simulink subsystem "acq_block"  (R2019b)
settings: Solver=VariableStepAuto  StartTime=0.0  StopTime=10.0  RelTol=1e-3
undefined symbols (not defined in the file): fs, Len, Radix
libraries: commseqgen3 x2, dspstat3 x2, dspsigops x2, dspxfrm3 x1
settings Model: Creator=nishantmittal  LastModifiedBy=nishantmittal

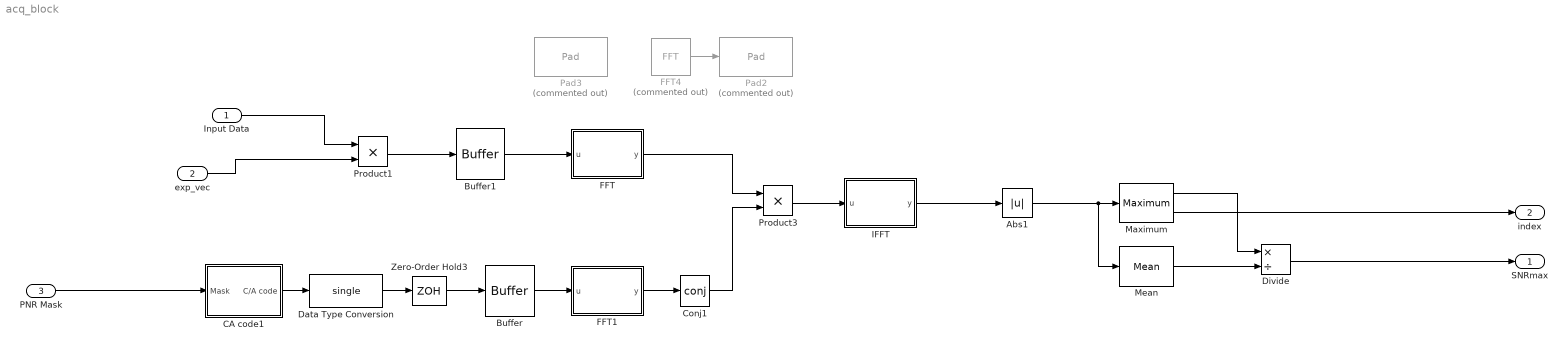
== system acq_block ==
  "Input Data " : Inport
  exp_vec : Inport  Port=2
  PNR Mask : Inport  Port=3
  Abs1 : Abs
  Buffer : Buffer  N=Len  ic=1  OutputFrames=off
  Buffer1 : Buffer  N=Len  ic=1  OutputFrames=off
  CA code1 : Subsystem
  Conj1 : Math  Operator=conj  SignedPower=off  SaturateOnIntegerOverflow=on
  Data Type Conversion : DataTypeConversion  OutDataTypeStr=single
  Divide : Product  Inputs=*/
  FFT : MATLAB Function  TreatAsAtomicUnit=on
  FFT1 : MATLAB Function  TreatAsAtomicUnit=on
  FFT4 : dspxfrm3/FFT  Commented=on  FFTImplementation=Radix-2  CompMethod=Table lookup  TableOpt=NEW  TableOptActive=Speed  BitRevOrder=off  Normalize=off  InheritFFTLength=off  FFTLength=2^15  WrapInput=on  roundingMode=Floor  overflowMode=off  firstCoeffDataTypeStr=Inherit: Same word length as input  firstCoeffLastDataTypeStr=Inherit: Same word length as input  outputMin=[]  outputMax=[]
  IFFT : MATLAB Function  TreatAsAtomicUnit=on
  Maximum : dspstat3/Maximum  operation=maximum  fcn=Value and Index  indexBase=One  operateOver=Each column  Dimension=1  InputProcessing=Columns as channels (frame based)  reset=None  roiEnable=off  roiType=Rectangles  roiPortion=Entire ROI  roiOutput=Individual statistics for each ROI  roiFlag=off  roundingMode=Floor  overflowMode=off  accumDataTypeStr=Inherit: Same as product output  accumLastDataTypeStr=Inherit: Same as product output
  Mean : dspstat3/Mean  run=off  InputProcessing=Columns as channels (frame based)  reset_popup=None  directionMode=Each column  dimension=1  roiEnable=off  roiType=Rectangles  roiPortion=Entire ROI  roiOutput=Individual statistics for each ROI  roiFlag=off  roundingMode=Floor  overflowMode=off  outputDataTypeStr=Inherit: Same as accumulator  outputMin=[]  outputMax=[]  outputLastDataTypeStr=Inherit: Same as accumulator
  Pad2 : dspsigops/Pad  Commented=on  padAlong=Columns  dimsToPad=1  valSrc=Specify via dialog  padVal=0  spec=Output size  padNumOutRowsSpecMethod=Next power of two  numOutRows=1  padNumOutColsSpecMethod=Next power of two  numOutCols=1  isVarDimsMode=off  padBeginning=0  padEnd=0  outSizeMode=User-specified  outSize=1  padSigAt=End  trunc_flag=None  roundingMode=Floor  overflowMode=off  truncOrWrapMode=Truncate  wrap_flag=None
      settings: SourceProductName=DSP System Toolbox  SourceProductBaseCode=DS
  Pad3 : dspsigops/Pad  Commented=on  padAlong=Columns  dimsToPad=1  valSrc=Specify via dialog  padVal=0  spec=Output size  padNumOutRowsSpecMethod=Next power of two  numOutRows=1  padNumOutColsSpecMethod=Next power of two  numOutCols=1  isVarDimsMode=off  padBeginning=0  padEnd=0  outSizeMode=User-specified  outSize=1  padSigAt=End  trunc_flag=None  roundingMode=Floor  overflowMode=off  truncOrWrapMode=Truncate  wrap_flag=None
      settings: SourceProductName=DSP System Toolbox  SourceProductBaseCode=DS
  Product1 : Product
  Product3 : Product
  Zero-Order Hold3 : ZeroOrderHold  SampleTime=1/fs
  SNRmax : Outport
  index : Outport  Port=2
  wires:
  Data Type Conversion/1 -> Zero-Order Hold3/1
  "Input Data "/1 -> Product1/1
  Product1/1 -> Buffer1/1
  Zero-Order Hold3/1 -> Buffer/1
  Abs1/1 -> Mean/1, Maximum/1
  CA code1/1(C/A code) -> Data Type Conversion/1
  PNR Mask/1 -> CA code1/1(Mask)
  exp_vec/1 -> Product1/2
  Maximum/1 -> Divide/1
  Mean/1 -> Divide/2
  Divide/1 -> SNRmax/1
  FFT4/1 -> Pad2/1
  Buffer1/1 -> FFT/1(u)
  Buffer/1 -> FFT1/1(u)
  FFT1/1(y) -> Conj1/1
  FFT/1(y) -> Product3/1
  Conj1/1 -> Product3/2
  Product3/1 -> IFFT/1(u)
  IFFT/1(y) -> Abs1/1
  Maximum/2 -> index/1

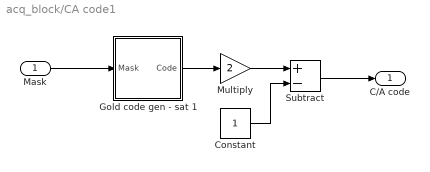
== system acq_block/CA code1 ==
  Mask : Inport
  Constant : Constant
  Gold code gen - sat 1 : Subsystem
  Multiply : Gain  Gain=2
  Subtract : Sum  Inputs=+-
  C/A code : Outport
  wires:
  Subtract/1 -> C/A code/1
  Multiply/1 -> Subtract/1
  Gold code gen - sat 1/1(Code) -> Multiply/1
  Constant/1 -> Subtract/2
  Mask/1 -> Gold code gen - sat 1/1(Mask)

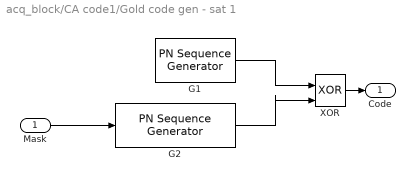
== system acq_block/CA code1/Gold code gen - sat 1 ==
  Mask : Inport
  G1 : commseqgen3/PN Sequence Generator  poly=[10 7 0]  ini_sta=[1 1 1 1 1 1 1 1 1 1]  outBitMaskSource=Dialog parameter  shift=[0 0 0 0 0 0 0 0 0 1]  outVarSiz=off  maxOutSizeMode=Dialog parameter  maxOutSize=[10 1]  Ts=1/(1.023e6)  sampPerFrame=1  reset=off  bitPackedOutputs=off  outDataType=boolean  numPackedBits=8  bitPackDataSigned=off  bitPackedOutDType=double
      settings: SourceProductName=Communications Toolbox
  G2 : commseqgen3/PN Sequence Generator  poly=[10 8 7 4 2 1 0]  ini_sta=[1 1 1 1 1 1 1 1 1 1]  outBitMaskSource=Input port  shift=[0 1 0 0 0 1 0 0 0 0]  outVarSiz=off  maxOutSizeMode=Dialog parameter  maxOutSize=[10 1]  Ts=1/(1.023e6)  sampPerFrame=1  reset=off  bitPackedOutputs=off  outDataType=boolean  numPackedBits=8  bitPackDataSigned=off  bitPackedOutDType=double
      settings: SourceProductName=Communications Toolbox
  XOR : Logic  Operator=XOR  IconShape=distinctive  AllPortsSameDT=off  OutDataTypeStr=boolean
  Code : Outport
  wires:
  G2/1 -> XOR/2
  XOR/1 -> Code/1
  G1/1 -> XOR/1
  Mask/1 -> G2/1

== matlab function acq_block/FFT ==
  data: u input; y output
function y = fcn(u)

y = fft(u);

== matlab function acq_block/FFT1 ==
  data: u input; y output
function y = fcn(u)

y = fft(u);

== matlab function acq_block/IFFT ==
  data: u input; y output
function y = fcn(u)

y = ifft(u);
